simulink model "reverb_mooer"  (R2024a)
settings: Solver=FixedStepAuto  StartTime=0.0  StopTime=10  RelTol=1e-3
values from neighbouring files (symbols this model uses):
  d1 = 5    [reverb_mooer_args.m]
  damp = 0.2    [reverb_mooer_args.m]
  Mix = 1    [reverb_mooer_args.m]
  Roomsize = 0.7    [reverb_mooer_args.m]
libraries: audiofeatures x3, dspvision x2, dspsnks4 x1
settings Model: Creator=fermata  LastModifiedBy=fermata

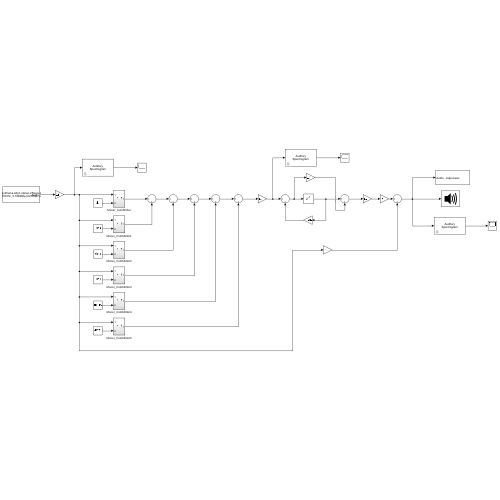
[thumbnail: Simulink's stored preview of the top-level diagram]
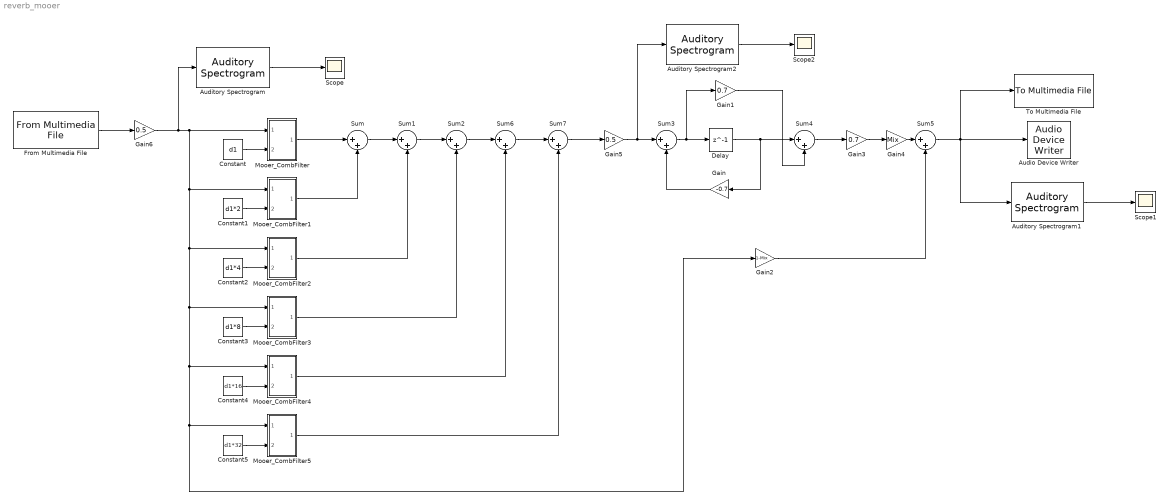
== system reverb_mooer ==
  Audio Device Writer : dspsnks4/Audio Device Writer  Driver=ALSA  Device=Default  InheritSampleRate=on  SampleRate=44100  BitDepth=16-bit integer  BufferSize=4096  NumBuffers=10  DefaultOutputChannelMapping=on  OutputChannelMapping=1:2  OutputNumUnderrunSamples=off  DriverIdx=8  DeviceWarnFlag=''
  Auditory Spectrogram : audiofeatures/Auditory Spectrogram  FrequencyScale=mel  MelStyle=oshaughnessy  AutoNumBands=on  NumBands=32  AutoFrequencyRange=on  FrequencyRange=[0, 22050]  FilterBankDesignDomain=linear  FilterBankNormalization=bandwidth  OutputFrequencyVector=off  WindowParameter=hamming(1024,'periodic')  WindowNormalization=on  OverlapLength=512  AutoFFTLength=on  FFTLength=1024  SpectrumType=magnitude  ApplyLog=off  NumHops=1  NumHopsOverlap=0  InheritSampleRate=off  SampleRate=44.1e3
  Auditory Spectrogram1 : audiofeatures/Auditory Spectrogram  FrequencyScale=mel  MelStyle=oshaughnessy  AutoNumBands=on  NumBands=32  AutoFrequencyRange=on  FrequencyRange=[0, 22050]  FilterBankDesignDomain=linear  FilterBankNormalization=bandwidth  OutputFrequencyVector=off  WindowParameter=hamming(1024,'periodic')  WindowNormalization=on  OverlapLength=512  AutoFFTLength=on  FFTLength=1024  SpectrumType=magnitude  ApplyLog=off  NumHops=1  NumHopsOverlap=0  InheritSampleRate=off  SampleRate=44.1e3
  Auditory Spectrogram2 : audiofeatures/Auditory Spectrogram  FrequencyScale=mel  MelStyle=oshaughnessy  AutoNumBands=on  NumBands=32  AutoFrequencyRange=on  FrequencyRange=[0, 22050]  FilterBankDesignDomain=linear  FilterBankNormalization=bandwidth  OutputFrequencyVector=off  WindowParameter=hamming(1024,'periodic')  WindowNormalization=on  OverlapLength=512  AutoFFTLength=on  FFTLength=1024  SpectrumType=magnitude  ApplyLog=off  NumHops=1  NumHopsOverlap=0  InheritSampleRate=off  SampleRate=44.1e3
  Constant : Constant  Value=d1
  Constant1 : Constant  Value=d1*2
  Constant2 : Constant  Value=d1*4
  Constant3 : Constant  Value=d1*8
  Constant4 : Constant  Value=d1*16
  Constant5 : Constant  Value=d1*32
  Delay : Delay  DelayLength=1  InitialCondition=0  UseCircularBuffer=on
  From Multimedia File : dspvision/From Multimedia File  inputFilename=/home/fermata/Development/Software/MATLAB/R2024a/toolbox/audio/samples/FunkyDrums-44p1-stereo-25secs.mp3  readRange=[1 Inf]  loop=on  numPlays=1  outputStreams=Audio only  videoDataType=single  audioDataType=double  inheritSampleTime=on  userDefinedSampleTime=1/1000  noAudioOutput=off  isIntensityVideo=off  fourcc=RGB  colorVideoFormat=Separate color signals  outputEOF=off  dataOrg=Column-major  audioFrameSize=1024  computeAudioFrameSize=off  outSamplingMode=Sample based
      settings: LibrarySourceBlock=audiosources/From Multimedia File
  Gain : Gain  Gain=-0.7
  Gain1 : Gain  Gain=0.7
  Gain2 : Gain  Gain=1-Mix
  Gain3 : Gain  Gain=0.7
  Gain4 : Gain  Gain=Mix
  Gain5 : Gain  Gain=0.5
  Gain6 : Gain  Gain=0.5
  Mooer_CombFilter : Subsystem
  Mooer_CombFilter1 : Subsystem
  Mooer_CombFilter2 : Subsystem
  Mooer_CombFilter3 : Subsystem
  Mooer_CombFilter4 : Subsystem
  Mooer_CombFilter5 : Subsystem
  Scope : Scope
  Scope1 : Scope
  Scope2 : Scope
  Sum{,1..2,6..7} (5 alike) : Sum  Inputs=|++  SaturateOnIntegerOverflow=on
  Sum3 : Sum  Inputs=|++
  Sum4 : Sum  Inputs=|++
  Sum5 : Sum  Inputs=|++
  To Multimedia File : dspvision/To Multimedia File  outputFilename=output.wav  streamSelection=Audio only  videoCompressor=None (uncompressed)  audioCompressor=None (uncompressed)  imagePorts=Separate color signals  fileType=WAV  audioDatatype=16-bit integer  fourcc=RGB  audioBitRate=128  audioQuality=75  videoQuality=75  mj2000CompFactor=10
      settings: LibrarySourceBlock=audiosinks/To Multimedia File
  wires:
  From Multimedia File/1 -> Gain6/1
  Auditory Spectrogram/1 -> Scope/1
  Auditory Spectrogram1/1 -> Scope1/1
  Constant/1 -> Mooer_CombFilter/2(In2)
  Constant1/1 -> Mooer_CombFilter1/2(In2)
  Constant2/1 -> Mooer_CombFilter2/2(In2)
  Constant3/1 -> Mooer_CombFilter3/2(In2)
  Sum/1 -> Sum1/1
  Sum1/1 -> Sum2/1
  Sum3/1 -> Delay/1, Gain1/1
  Delay/1 -> Sum4/1, Gain/1
  Sum4/1 -> Gain3/1
  Mooer_CombFilter1/1(Out1) -> Sum/2
  Mooer_CombFilter2/1(Out1) -> Sum1/2
  Mooer_CombFilter/1(Out1) -> Sum/1
  Auditory Spectrogram2/1 -> Scope2/1
  Sum5/1 -> To Multimedia File/1, Auditory Spectrogram1/1, Audio Device Writer/1
  Gain2/1 -> Sum5/2
  Gain3/1 -> Gain4/1
  Gain4/1 -> Sum5/1
  Mooer_CombFilter3/1(Out1) -> Sum2/2
  Gain5/1 -> Auditory Spectrogram2/1, Sum3/1
  Constant4/1 -> Mooer_CombFilter4/2(In2)
  Constant5/1 -> Mooer_CombFilter5/2(In2)
  Mooer_CombFilter5/1(Out1) -> Sum7/2
  Mooer_CombFilter4/1(Out1) -> Sum6/2
  Gain/1 -> Sum3/2
  Gain1/1 -> Sum4/2
  Sum2/1 -> Sum6/1
  Sum6/1 -> Sum7/1
  Sum7/1 -> Gain5/1
  Gain6/1 -> Auditory Spectrogram/1, Mooer_CombFilter/1(In1), Mooer_CombFilter1/1(In1), Mooer_CombFilter2/1(In1), Mooer_CombFilter3/1(In1), Mooer_CombFilter4/1(In1), Mooer_CombFilter5/1(In1), Gain2/1

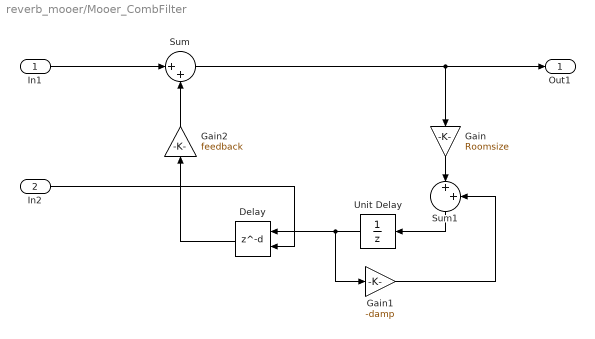
== system reverb_mooer/Mooer_CombFilter ==
  In1 : Inport
  In2 : Inport  Port=2
  Delay : Delay  DelayLengthSource=Input port  DelayLength=10  InitialCondition=0
      settings: InputPortMap=u0,p1
  Gain : Gain  Gain=Roomsize  SaturateOnIntegerOverflow=on
  Gain1 : Gain  Gain=-damp
  Gain2 : Gain  Gain=feedback
  Sum : Sum  Inputs=|++  SaturateOnIntegerOverflow=on
  Sum1 : Sum  Inputs=|++
  Unit Delay : UnitDelay  SampleTime=-1  HasFrameUpgradeWarning=on
  Out1 : Outport
  wires:
  Gain1/1 -> Sum1/2
  Gain/1 -> Sum1/1
  In1/1 -> Sum/1
  Unit Delay/1 -> Gain1/1, Delay/1
  Sum1/1 -> Unit Delay/1
  Sum/1 -> Out1/1, Gain/1
  In2/1 -> Delay/2
  Delay/1 -> Gain2/1
  Gain2/1 -> Sum/2

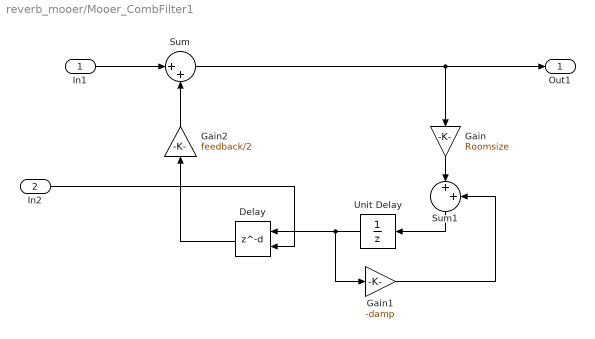
== system reverb_mooer/Mooer_CombFilter1 ==
  In1 : Inport
  In2 : Inport  Port=2
  Delay : Delay  DelayLengthSource=Input port  DelayLength=10  InitialCondition=0
      settings: InputPortMap=u0,p1
  Gain : Gain  Gain=Roomsize  SaturateOnIntegerOverflow=on
  Gain1 : Gain  Gain=-damp
  Gain2 : Gain  Gain=feedback/2
  Sum : Sum  Inputs=|++  SaturateOnIntegerOverflow=on
  Sum1 : Sum  Inputs=|++
  Unit Delay : UnitDelay  SampleTime=-1  HasFrameUpgradeWarning=on
  Out1 : Outport
  wires:
  Gain1/1 -> Sum1/2
  Gain/1 -> Sum1/1
  In1/1 -> Sum/1
  Unit Delay/1 -> Gain1/1, Delay/1
  Sum1/1 -> Unit Delay/1
  Sum/1 -> Out1/1, Gain/1
  In2/1 -> Delay/2
  Delay/1 -> Gain2/1
  Gain2/1 -> Sum/2

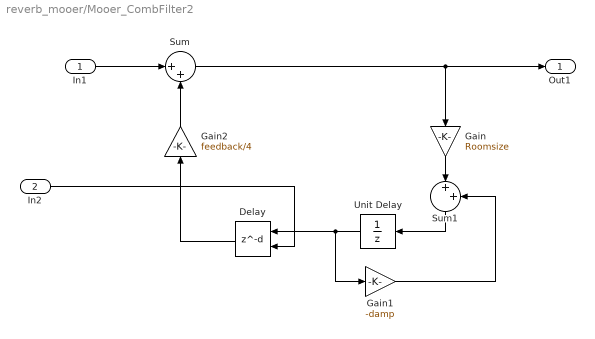
== system reverb_mooer/Mooer_CombFilter2 ==
  In1 : Inport
  In2 : Inport  Port=2
  Delay : Delay  DelayLengthSource=Input port  DelayLength=10  InitialCondition=0
      settings: InputPortMap=u0,p1
  Gain : Gain  Gain=Roomsize  SaturateOnIntegerOverflow=on
  Gain1 : Gain  Gain=-damp
  Gain2 : Gain  Gain=feedback/4
  Sum : Sum  Inputs=|++  SaturateOnIntegerOverflow=on
  Sum1 : Sum  Inputs=|++
  Unit Delay : UnitDelay  SampleTime=-1  HasFrameUpgradeWarning=on
  Out1 : Outport
  wires:
  Gain1/1 -> Sum1/2
  Gain/1 -> Sum1/1
  In1/1 -> Sum/1
  Unit Delay/1 -> Gain1/1, Delay/1
  Sum1/1 -> Unit Delay/1
  Sum/1 -> Out1/1, Gain/1
  In2/1 -> Delay/2
  Delay/1 -> Gain2/1
  Gain2/1 -> Sum/2

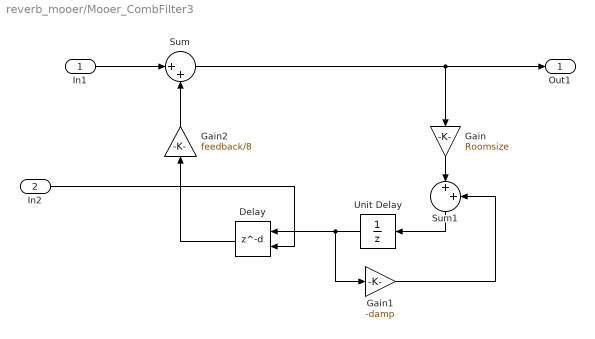
== system reverb_mooer/Mooer_CombFilter3 ==
  In1 : Inport
  In2 : Inport  Port=2
  Delay : Delay  DelayLengthSource=Input port  DelayLength=10  InitialCondition=0
      settings: InputPortMap=u0,p1
  Gain : Gain  Gain=Roomsize  SaturateOnIntegerOverflow=on
  Gain1 : Gain  Gain=-damp
  Gain2 : Gain  Gain=feedback/8
  Sum : Sum  Inputs=|++  SaturateOnIntegerOverflow=on
  Sum1 : Sum  Inputs=|++
  Unit Delay : UnitDelay  SampleTime=-1  HasFrameUpgradeWarning=on
  Out1 : Outport
  wires:
  Gain1/1 -> Sum1/2
  Gain/1 -> Sum1/1
  In1/1 -> Sum/1
  Unit Delay/1 -> Gain1/1, Delay/1
  Sum1/1 -> Unit Delay/1
  Sum/1 -> Out1/1, Gain/1
  In2/1 -> Delay/2
  Delay/1 -> Gain2/1
  Gain2/1 -> Sum/2

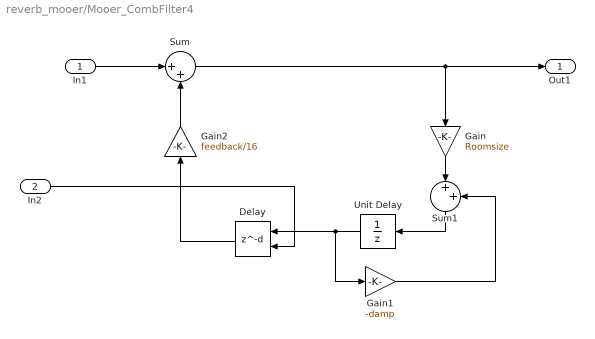
== system reverb_mooer/Mooer_CombFilter4 ==
  In1 : Inport
  In2 : Inport  Port=2
  Delay : Delay  DelayLengthSource=Input port  DelayLength=10  InitialCondition=0
      settings: InputPortMap=u0,p1
  Gain : Gain  Gain=Roomsize  SaturateOnIntegerOverflow=on
  Gain1 : Gain  Gain=-damp
  Gain2 : Gain  Gain=feedback/16
  Sum : Sum  Inputs=|++  SaturateOnIntegerOverflow=on
  Sum1 : Sum  Inputs=|++
  Unit Delay : UnitDelay  SampleTime=-1  HasFrameUpgradeWarning=on
  Out1 : Outport
  wires:
  Gain1/1 -> Sum1/2
  Gain/1 -> Sum1/1
  In1/1 -> Sum/1
  Unit Delay/1 -> Gain1/1, Delay/1
  Sum1/1 -> Unit Delay/1
  Sum/1 -> Out1/1, Gain/1
  In2/1 -> Delay/2
  Delay/1 -> Gain2/1
  Gain2/1 -> Sum/2

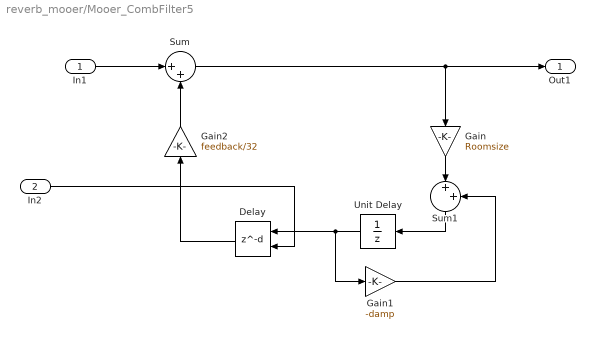
== system reverb_mooer/Mooer_CombFilter5 ==
  In1 : Inport
  In2 : Inport  Port=2
  Delay : Delay  DelayLengthSource=Input port  DelayLength=10  InitialCondition=0
      settings: InputPortMap=u0,p1
  Gain : Gain  Gain=Roomsize  SaturateOnIntegerOverflow=on
  Gain1 : Gain  Gain=-damp
  Gain2 : Gain  Gain=feedback/32
  Sum : Sum  Inputs=|++  SaturateOnIntegerOverflow=on
  Sum1 : Sum  Inputs=|++
  Unit Delay : UnitDelay  SampleTime=-1  HasFrameUpgradeWarning=on
  Out1 : Outport
  wires:
  Gain1/1 -> Sum1/2
  Gain/1 -> Sum1/1
  In1/1 -> Sum/1
  Unit Delay/1 -> Gain1/1, Delay/1
  Sum1/1 -> Unit Delay/1
  Sum/1 -> Out1/1, Gain/1
  In2/1 -> Delay/2
  Delay/1 -> Gain2/1
  Gain2/1 -> Sum/2
